simulink model "nco_lut_direct_quarter"  (R2016a)
settings: Solver=VariableStepAuto  StartTime=0.0  StopTime=10.0  RelTol=1e-3
libraries: hdlsllib x3, simulink x3
settings Model: Creator=sj660  LastModifiedBy=sj660

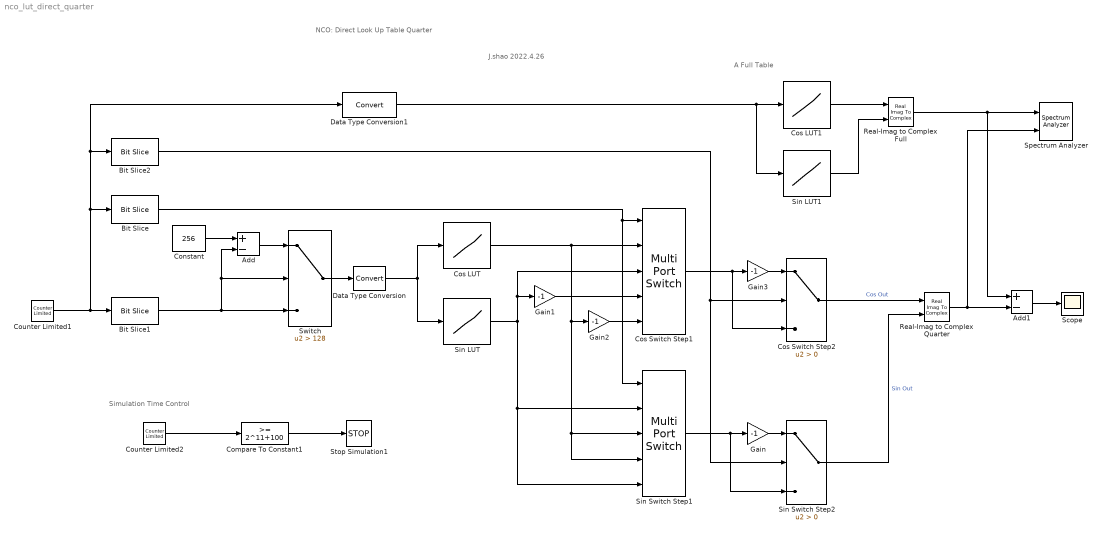
== system nco_lut_direct_quarter ==
  note: A Full Table
  note: NCO: Direct Look Up Table Quarter
  note: J.shao 2022.4.26
  note: Simulation Time Control
  Add : Sum  Inputs=+-
  Add1 : Sum  Inputs=+-
  Bit Slice : hdlsllib/HDL Operations/Bit Slice  lidx=8  ridx=7
  Bit Slice1 : hdlsllib/HDL Operations/Bit Slice  lidx=7  ridx=0
  Bit Slice2 : hdlsllib/HDL Operations/Bit Slice  lidx=9  ridx=9
  Compare To Constant1 : simulink/Logic and Bit Operations/Compare To Constant  relop=>=  const=2^11+100  OutDataTypeStr=boolean
  Constant : Constant  Value=256
  Cos LUT : Lookup_n-D  NumberOfTableDimensions=1  BreakpointsForDimension1=[0:1:128]  BreakpointsForDimension1FirstPoint=0  UseOneInputPortForAllInputData=on  Table=cos([0:2*pi/1024:pi/4])  InterpMethod=Nearest  ExtrapMethod=Cubic spline  InternalRulePriority=Speed  OutDataTypeStr=fixdt(1,13,11)  RndMeth=Simplest  InputSameDT=on
  Cos LUT1 : Lookup_n-D  NumberOfTableDimensions=1  BreakpointsForDimension1=[0:1:1023]  BreakpointsForDimension1FirstPoint=0  UseOneInputPortForAllInputData=on  Table=cos([0:2*pi/1024:2*pi-2*pi/1024])  InterpMethod=Nearest  ExtrapMethod=Cubic spline  InternalRulePriority=Speed  OutDataTypeStr=fixdt(1,13,11)  RndMeth=Simplest  InputSameDT=on
  Cos Switch Step1 : MultiPortSwitch  DataPortOrder=Zero-based contiguous  Inputs=4  DiagnosticForDefault=None
  Cos Switch Step2 : Switch  Criteria=u2 > Threshold
  Counter Limited1 : simulink/Sources/Counter Limited  uplimit=2^10-1  tsamp=1e-9
  Counter Limited2 : simulink/Sources/Counter Limited  uplimit=2^12  tsamp=1e-9
  Data Type Conversion : DataTypeConversion
  Data Type Conversion1 : DataTypeConversion
  Gain : Gain  Gain=-1
  Gain1 : Gain  Gain=-1
  Gain2 : Gain  Gain=-1
  Gain3 : Gain  Gain=-1  OutDataTypeStr=Inherit: Same as input
  Real-Imag to Complex Full : RealImagToComplex
  Real-Imag to Complex Quarter : RealImagToComplex
  Scope : Scope
  Sin LUT : Lookup_n-D  NumberOfTableDimensions=1  BreakpointsForDimension1=[0:1:128]  BreakpointsForDimension1FirstPoint=0  UseOneInputPortForAllInputData=on  Table=sin([0:2*pi/1024:pi/4])  InterpMethod=Nearest  ExtrapMethod=Cubic spline  InternalRulePriority=Speed  OutDataTypeStr=fixdt(1,13,11)  RndMeth=Simplest  InputSameDT=on
  Sin LUT1 : Lookup_n-D  NumberOfTableDimensions=1  BreakpointsForDimension1=[0:1:1023]  BreakpointsForDimension1FirstPoint=0  UseOneInputPortForAllInputData=on  Table=sin([0:2*pi/1024:2*pi-2*pi/1024])  InterpMethod=Nearest  ExtrapMethod=Cubic spline  InternalRulePriority=Speed  OutDataTypeStr=fixdt(1,13,11)  RndMeth=Simplest  InputSameDT=on
  Sin Switch Step1 : MultiPortSwitch  DataPortOrder=Zero-based contiguous  Inputs=4  DiagnosticForDefault=None
  Sin Switch Step2 : Switch  Criteria=u2 > Threshold
  Spectrum Analyzer : SpectrumAnalyzer  NumInputPorts=2
  Stop Simulation1 : Stop
  Switch : Switch  Criteria=u2 > Threshold  Threshold=128
  wires:
  Counter Limited1/1 -> Data Type Conversion1/1, Bit Slice2/1, Bit Slice/1, Bit Slice1/1
  Data Type Conversion/1 -> Cos LUT/1, Sin LUT/1
  Cos LUT/1 -> Sin Switch Step1/4, Sin Switch Step1/3, Gain2/1, Cos Switch Step1/2
  Sin LUT/1 -> Gain1/1, Cos Switch Step1/3, Sin Switch Step1/5, Sin Switch Step1/2
  Counter Limited2/1 -> Compare To Constant1/1
  Compare To Constant1/1 -> Stop Simulation1/1
  Bit Slice1/1 -> Add/2, Switch/2, Switch/3
  Switch/1 -> Data Type Conversion/1
  Add/1 -> Switch/1
  Constant/1 -> Add/1
  Bit Slice/1 -> Cos Switch Step1/1, Sin Switch Step1/1
  Bit Slice2/1 -> Sin Switch Step2/2, Cos Switch Step2/2
  Sin Switch Step1/1 -> Gain/1, Sin Switch Step2/3
  Gain/1 -> Sin Switch Step2/1
  Gain1/1 -> Cos Switch Step1/4
  Gain2/1 -> Cos Switch Step1/5
  Cos Switch Step1/1 -> Cos Switch Step2/3, Gain3/1
  Sin Switch Step2/1 -> Real-Imag to Complex Quarter/2  "Sin Out"
  Cos Switch Step2/1 -> Real-Imag to Complex Quarter/1  "Cos Out"
  Gain3/1 -> Cos Switch Step2/1
  Data Type Conversion1/1 -> Cos LUT1/1, Sin LUT1/1
  Cos LUT1/1 -> Real-Imag to Complex Full/1
  Sin LUT1/1 -> Real-Imag to Complex Full/2
  Real-Imag to Complex Quarter/1 -> Add1/2, Spectrum Analyzer/2
  Real-Imag to Complex Full/1 -> Spectrum Analyzer/1, Add1/1
  Add1/1 -> Scope/1
